simulink subsystem "SD_Filter"  (R2020b)
settings: Solver=VariableStepAuto  StartTime=0.0  StopTime=10.0  RelTol=1e-3
values from neighbouring files (symbols this model uses):
  alpha = den_ts    [sd_filter_top.m]
  beta = num_ts    [sd_filter_top.m]
  ts = 1/fs    (= 8.85770975057e-08)    [sd_2nd_mod.m]    (also in sd_2nd_mod_top.m; sd_filter_top.m)
undefined symbols (not defined in the file or in its folder): k
settings Model: Creator=1111293  LastModifiedBy=1111293

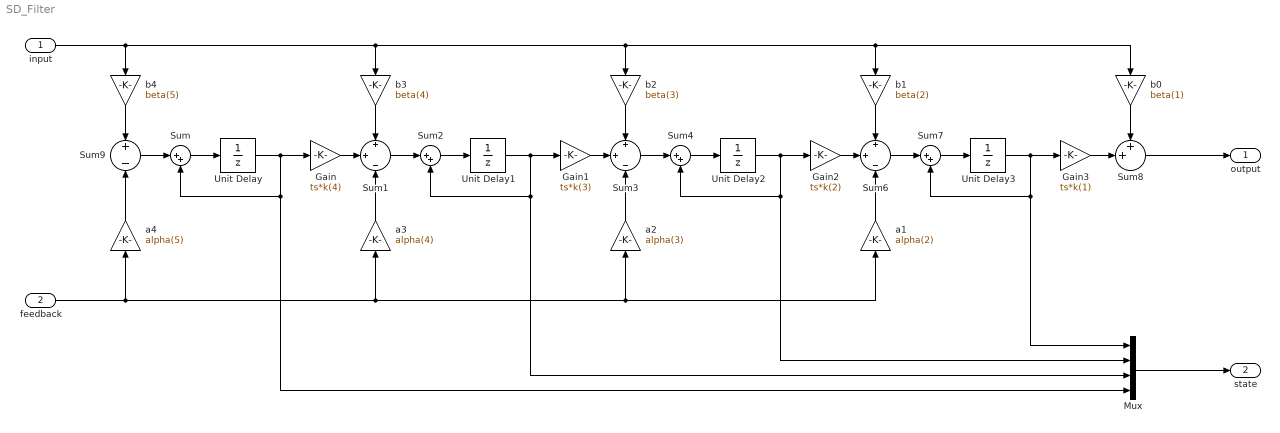
== system SD_Filter ==
  input : Inport
  feedback : Inport  Port=2
  Gain : Gain  Gain=ts*k(4)  RndMeth=Round
  Gain1 : Gain  Gain=ts*k(3)  RndMeth=Round
  Gain2 : Gain  Gain=ts*k(2)  RndMeth=Round
  Gain3 : Gain  Gain=ts*k(1)  RndMeth=Round
  Mux : Mux
  Sum{,2,4,7} (4 alike) : Sum  Inputs=|++
  Sum1 : Sum  Inputs=+|+|-
  Sum3 : Sum  Inputs=+|+|-
  Sum6 : Sum  Inputs=+|+|-
  Sum8 : Sum  Inputs=++|
  Sum9 : Sum  Inputs=+|-
  Unit Delay{,1..3} (4 alike) : UnitDelay  SampleTime=-1  HasFrameUpgradeWarning=on
  a1 : Gain  Gain=alpha(2)
  a2 : Gain  Gain=alpha(3)
  a3 : Gain  Gain=alpha(4)
  a4 : Gain  Gain=alpha(5)
  b0 : Gain  Gain=beta(1)
  b1 : Gain  Gain=beta(2)
  b2 : Gain  Gain=beta(3)
  b3 : Gain  Gain=beta(4)
  b4 : Gain  Gain=beta(5)
  output : Outport
  state : Outport  Port=2
  wires:
  Unit Delay3/1 -> Gain3/1, Sum7/2, Mux/1
  Sum3/1 -> Sum4/1
  Unit Delay2/1 -> Gain2/1, Sum4/2, Mux/2
  Sum2/1 -> Unit Delay1/1
  Gain/1 -> Sum1/2
  b3/1 -> Sum1/1
  Sum6/1 -> Sum7/1
  feedback/1 -> a1/1, a2/1, a3/1, a4/1
  Unit Delay1/1 -> Gain1/1, Sum2/2, Mux/3
  b2/1 -> Sum3/1
  input/1 -> b4/1, b3/1, b2/1, b1/1, b0/1
  Gain2/1 -> Sum6/2
  b0/1 -> Sum8/1
  Sum9/1 -> Sum/1
  Sum4/1 -> Unit Delay2/1
  Sum8/1 -> output/1
  Sum7/1 -> Unit Delay3/1
  Mux/1 -> state/1
  a3/1 -> Sum1/3
  Gain1/1 -> Sum3/2
  a2/1 -> Sum3/3
  a4/1 -> Sum9/2
  b4/1 -> Sum9/1
  a1/1 -> Sum6/3
  Unit Delay/1 -> Gain/1, Sum/2, Mux/4
  Sum/1 -> Unit Delay/1
  Sum1/1 -> Sum2/1
  Gain3/1 -> Sum8/2
  b1/1 -> Sum6/1
